simulink model "rtwdemo_sil_topmodel"  (Simulink 7.6)
settings: Solver=FixedStepDiscrete  StartTime=0.0  StopTime=10.0  FixedStep=T  RelTol=1e-3
model workspace (MAT data in the model file):
  myUpper : Simulink.Parameter (value not decoded)
  myLower : Simulink.Parameter (value not decoded)
PostLoadFcn:
  | rtwdemo_overrides='{''LaunchReport'',''PassReuseOutputArgsAs''}';
  | rtwconfiguredemo(gcs,'fixed',false,rtwdemo_overrides);
  | clear rtwdemo_overrides
  | 
  | % Sample time
  | T=0.1;
  | [ticks_to_count, reset] = rtwdemo_sil_topmodel_data(T);
Description:
  | Example model reference component.
settings Model: Creator=The MathWorks Inc.  SimulationMode=software-in-the-loop (sil)  ExtModeAutoUpdateStatusClock=off
settings DataIOCC: ExternalInput=ticks_to_count, reset  LimitDataPoints=off  LoadExternalInput=on  SaveFormat=StructureWithTime  SaveOutput=off  SaveTime=off  ReturnWorkspaceOutputs=on  SignalLoggingName=logsOut
settings OptimizationCC: InlineParams=on  UseIntDivNetSlope=on  InlineInvariantSignals=on  EnhancedBackFolding=on  BooleansAsBitfields=on  PassReuseOutputArgsAs=Individual arguments  StateBitsets=on  DataBitsets=on  UseTempVars=on  ZeroExternalMemoryAtStartup=off  ZeroInternalMemoryAtStartup=off  NoFixptDivByZeroProtection=on  EfficientFloat2IntCast=on  OptimizeModelRefInitCode=on  LifeSpan=1  SimCompilerOptimization=On
settings DebuggingCC: UnderspecifiedInitializationDetection=Simplified  MergeDetectMultiDrivingBlocksExec=error  CheckExecutionContextPreStartOutputMsg=on  CheckExecutionContextRuntimeOutputMsg=on  SolverPrmCheckMsg=none  UniqueDataStoreMsg=error  ModelReferenceSymbolNameMessage=none  StrictBusMsg=ErrorOnBusTreatedAsVector
settings HardwareCC: ProdIntDivRoundTo=Zero  ProdEndianess=LittleEndian  ProdHWDeviceType=Specified  TargetHWDeviceType=Generic->32-bit Embedded Processor
settings ModelReferenceCC: CheckModelReferenceTargetMessage=none  ModelReferencePassRootInputsByReference=off
settings RTWCC: SystemTargetFile=ert.tlc  TLCOptions=-p0 -aWarnNonSaturatedBlocks=0  TemplateMakefile=ert_default_tmf  Description=Real-Time Workshop Embedded Coder  GenerateReport=on  RTWVerbose=off  ProcessScript=ert_make_rtw_hook  IncludeHyperlinkInReport=on  GenerateTraceInfo=on  GenerateTraceReport=on  GenerateTraceReportSl=on  GenerateTraceReportSf=on  GenerateTraceReportEml=on
settings CodeAppCC: ForceParamTrailComments=on  IgnoreCustomStorageClasses=off  IgnoreTestpoints=on  SimulinkDataObjDesc=on  CustomSymbolStrGlobalVar=rt$N$M  CustomSymbolStrType=$N$M  CustomSymbolStrFcn=$N$M$F  CustomSymbolStrMacro=$N$M  InsertBlockDesc=on
settings ERTTargetCC: MultiwordLength=2048  GenerateSampleERTMain=on  IncludeMdlTerminateFcn=off  CombineSignalStateStructs=on  SupportNonFinite=off  SupportComplex=off  PurelyIntegerCode=on  InlinedParameterPlacement=NonHierarchical  ERTCustomFileTemplate=example_file_process.tlc  ERTFilePackagingFormat=CompactWithDataFile  ConvertIfToSwitch=off

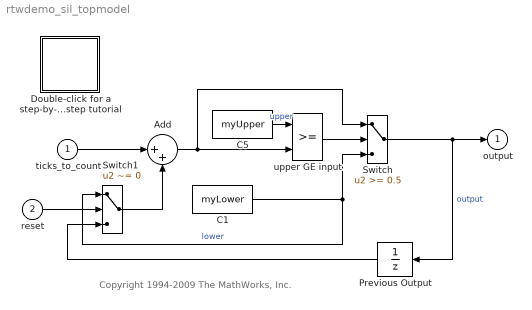
== system rtwdemo_sil_topmodel ==
  note: Copyright 1994-2009 The MathWorks, Inc.
  " ticks_to_count" : Inport  OutDataTypeStr=boolean  PortDimensions=1  SampleTime=T
  reset : Inport  Port=2  OutDataTypeStr=boolean  PortDimensions=1  SampleTime=T
  Add : Sum  Inputs=|++  OutDataTypeStr=uint8
  C1 : Constant  Value=myLower  OutDataTypeStr=uint8
  C5 : Constant  Value=myUpper  OutDataTypeStr=uint8
  Double-click for a step-by-step tutorial : Subsystem
      settings: OpenFcn=showdemo('rtwdemo_sil_pil_script');
      mask Type: Info
      mask Display: image(imread('targets_demo_info.bmp','bmp'),'center')
  Previous Output : UnitDelay  X0=50  SampleTime=T
  Switch : Switch  Threshold=0.5  InputSameDT=on
  Switch1 : Switch  Criteria=u2 ~= 0  Threshold=0.5  InputSameDT=on
  upper GE input : RelationalOperator  Priority=0  InputSameDT=on
      settings: AttributesFormatString=\n
  output : Outport
  wires:
  Switch/1 -> output/1, Previous Output/1  "output"
  upper GE input/1 -> Switch/2
  C5/1 -> upper GE input/1  "upper"
  Add/1 -> upper GE input/2, Switch/1
  C1/1 -> Switch/3, Switch1/1  "lower"
  " ticks_to_count"/1 -> Add/1
  reset/1 -> Switch1/2
  Previous Output/1 -> Switch1/3
  Switch1/1 -> Add/2

== system rtwdemo_sil_topmodel/Double-click for a step-by-step tutorial ==
